simulink subsystem "PieroAJ_ModelZ"  (R2023b)
settings: Solver=VariableStepAuto  StartTime=0.0  StopTime=10.0  RelTol=1e-3
settings Model: Creator=USUARIO  LastModifiedBy=USUARIO

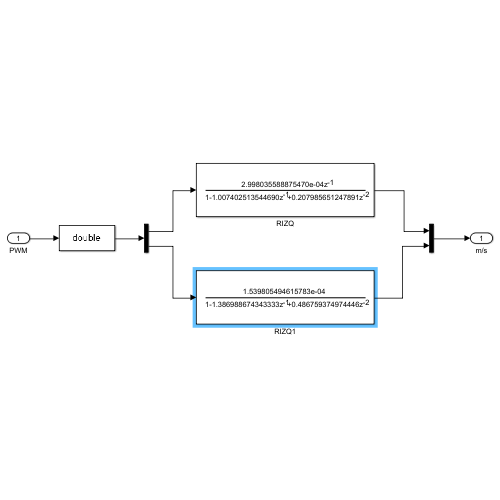
[thumbnail: Simulink's stored preview of the top-level diagram]
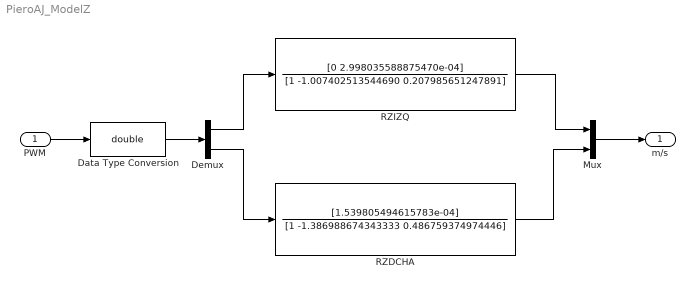
== system PieroAJ_ModelZ ==
  PWM : Inport
  Data Type Conversion : DataTypeConversion  OutDataTypeStr=double  SaturateOnIntegerOverflow=off  RndMeth=Floor
  Demux : Demux  Outputs=2
  Mux : Mux  Inputs=2
  RZDCHA : DiscreteFilter  Numerator=[1.539805494615783e-04]  Denominator=[1 -1.386988674343333 0.486759374974446]
  RZIZQ : DiscreteFilter  Numerator=[0 2.998035588875470e-04]  Denominator=[1 -1.007402513544690 0.207985651247891]
  m/s : Outport
  wires:
  Demux/2 -> RZDCHA/1
  RZDCHA/1 -> Mux/2
  RZIZQ/1 -> Mux/1
  Demux/1 -> RZIZQ/1
  Mux/1 -> m/s/1
  Data Type Conversion/1 -> Demux/1
  PWM/1 -> Data Type Conversion/1
